simulink model "main"  (R2019a)
settings: Solver=ode45  StartTime=0.0  StopTime=simTime  FixedStep=Ts  RelTol=1e-3  EnableMultiTasking=on
values from neighbouring files (symbols this model uses):
  alfa1 = .2    (= 0.2)    [parameters.m]
  alfa2 = .2    (= 0.2)    [parameters.m]
  b1 = 0.1    [parameters.m]
  b2 = 0.1    [parameters.m]
  b3_nom = 0.1    [parameters.m]
  b4_nom = 0.1    [parameters.m]
  b5 = 0.1    [parameters.m]
  C = zeros(2,10); C(1,1) = 1; C(2,4) = 1    [parameters.m]
  C_D_Re_GNARC = C_C_Re    [init.m]
  D_D_Re_GNARC = D_C_Re    [init.m]
  DELTAS = cat(3,DELTAS,delta_c2d)    [dht.m]
  GAMMA = eye(10)    [parameters.m]
  initial_P = inmat.P_ss    [parameters.m]
  initial_probs = [1.0/N_hypos 1.0/N_hypos 1.0/N_hypos]    [dht.m]
  initial_state = [0,0,0,0,0,0,0,0,0,0]'    [parameters.m]
  k1 = 0.15    [parameters.m]
  k2 = (2.5-0.75)/2    (= 0.875)    [parameters.m]
  k3_nom = .1    (= 0.1)    [parameters.m]
  k4_nom = .1    (= 0.1)    [parameters.m]
  k5 = (2.5-0.9)/2    (= 0.8)    [parameters.m]
  Ks = cat(3,Ks,Li)    [dht.m]
  ks = [[2.0 2.0]; [1.0 1.75]; [2.0 1.25]]    [dht.m]
  m1 = 1    [parameters.m]
  m2 = 1    [parameters.m]
  m3 = 1    [parameters.m]
  m4 = 1    [parameters.m]
  PHIS = cat(3,PHIS,phi_c2d)    [dht.m]
  Qd = A_d*N(1:10, 11:20)    [parameters.m]
  Rd = R ./ Ts    [parameters.m]
  Sh_dets = cat(3,Sh_dets,det(Shtemp))    [dht.m]
  Sh_invs = cat(3,Sh_invs,inv(Shtemp))    [dht.m]
  simNo = 10    [parameters.m]    (also in qsimall.m = i)
  simTime = 300    [parameters.m]    (also in qsimall.m = 400)
  Ts = .001    (= 0.001)    [parameters.m]
undefined symbols (not defined in the file or in its folder): A_D_Re_GNARC, B_D_Re_GNARC, DELTA, PHI
libraries: simulink x4
settings Model: Creator=VAHiD  LastModifiedBy=revolt
settings DataIOCC: LimitDataPoints=on  SaveFormat=Array  SignalLoggingSaveFormat=ModelDataLogs  ReturnWorkspaceOutputs=off
settings OptimizationCC: ExpressionDepthLimit=2147483647  LifeSpan=inf
settings DebuggingCC: UnderspecifiedInitializationDetection=Classic  MergeDetectMultiDrivingBlocksExec=none  SolverPrmCheckMsg=warning  FcnCallInpInsideContextMsg=warning  StateNameClashWarn=warning  PregeneratedLibrarySubsystemCodeDiagnostic=none  SFUnexpectedBacktrackingDiag=warning  SFNoUnconditionalDefaultTransitionDiag=warning  SFExecutionAtInitializationDiag=none  ArithmeticOperatorsInVariantConditions=warning
settings HardwareCC: ProdBitPerPointer=32  ProdBitPerSizeT=32  ProdBitPerPtrDiffT=32  ProdLargestAtomicFloat=None  ProdIntDivRoundTo=Undefined  ProdEndianess=Unspecified  ProdWordSize=32  ProdHWDeviceType=32-bit Generic
settings ModelReferenceCC: PropagateSignalLabelsOutOfModel=off
settings SFSimCC: SimUseLocalCustomCode=off
settings RTWCC: RTWUseLocalCustomCode=off
settings CodeAppCC: StateflowObjectComments=on
settings GRTTargetCC: TargetLangStandard=C89/C90 (ANSI)  GeneratePreprocessorConditionals=Disable all  CombineOutputUpdateFcns=off  GRTInterface=on
settings ConfigComp: CovMetricSettings=dw  CovHtmlReporting=on  CovSaveCumulativeToWorkspaceVar=on  CovSaveSingleToWorkspaceVar=on  CovExternalEMLEnable=off

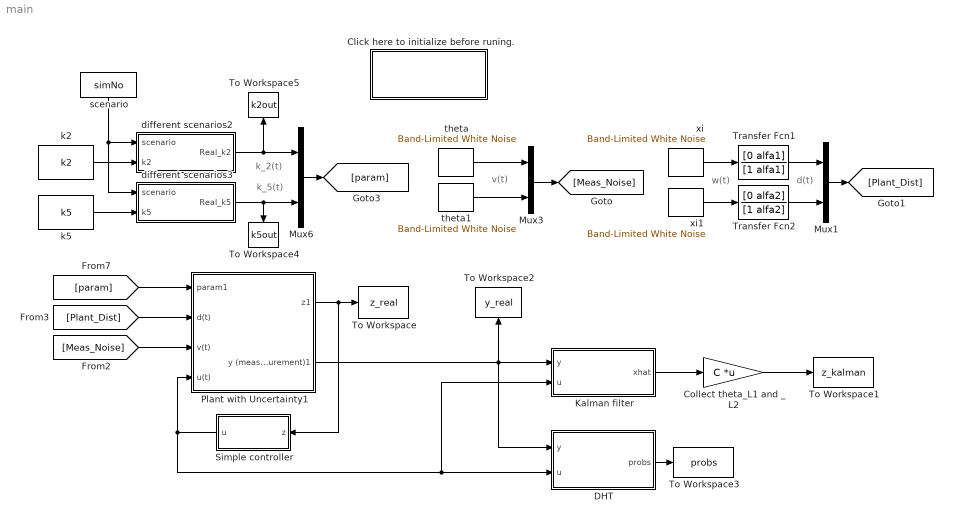
== system main ==
  note: w(t)
  note: v(t)
  note: d(t)
  note: k_2(t)
  note: k_5(t)
  Click here to initialize before runing. : Subsystem
      settings: OpenFcn=start_up
      mask Display: disp('Load\Parameters')
  Collect theta_L1 and _L2 : Gain  Gain=C  Multiplication=Matrix(K*u)
  DHT : Subsystem
  Kalman filter : Subsystem
  Mux1 : Mux  Inputs=2
  Mux3 : Mux  Inputs=2
  Mux6 : Mux  Inputs=2
  Plant with Uncertainty1 : Subsystem
  Simple controller : Subsystem
  To Workspace : ToWorkspace  VariableName=z_real  SaveFormat=Timeseries  SampleTime=-1
  To Workspace1 : ToWorkspace  VariableName=z_kalman  SaveFormat=Timeseries  SampleTime=-1
  To Workspace2 : ToWorkspace  VariableName=y_real  SaveFormat=Timeseries  SampleTime=-1
  To Workspace3 : ToWorkspace  VariableName=probs  SaveFormat=Timeseries  SampleTime=-1
  To Workspace4 : ToWorkspace  VariableName=k5out  SaveFormat=Timeseries  SampleTime=-1
  To Workspace5 : ToWorkspace  VariableName=k2out  SaveFormat=Timeseries  SampleTime=-1
  Transfer Fcn1 : TransferFcn  Numerator=[0 alfa1]  Denominator=[1 alfa1]
  Transfer Fcn2 : TransferFcn  Numerator=[0 alfa2]  Denominator=[1 alfa2]
  different scenarios2 : Subsystem
  different scenarios3 : Subsystem
  k2 : Constant  Value=k2
  k5 : Constant  Value=k5
  scenario : Constant  Value=simNo
  theta : simulink/Sources/Band-Limited White Noise  Cov=TH1  Ts=Ts  seed=1
  theta1 : simulink/Sources/Band-Limited White Noise  Cov=TH2  Ts=Ts  seed=2
  xi : simulink/Sources/Band-Limited White Noise  Cov=XI1  Ts=Ts  seed=3
  xi1 : simulink/Sources/Band-Limited White Noise  Cov=XI2  Ts=Ts  seed=4
  wires:
  Mux3/1 -> [Meas_Noise]
  theta/1 -> Mux3/1
  theta1/1 -> Mux3/2
  Mux1/1 -> [Plant_Dist]
  xi/1 -> Transfer Fcn1/1
  xi1/1 -> Transfer Fcn2/1
  Transfer Fcn1/1 -> Mux1/1
  Transfer Fcn2/1 -> Mux1/2
  scenario/1 -> different scenarios2/1(scenario), different scenarios3/1(scenario)
  k2/1 -> different scenarios2/2(k2)
  k5/1 -> different scenarios3/2(k5)
  different scenarios3/1(Real_k5) -> Mux6/2, To Workspace4/1
  different scenarios2/1(Real_k2) -> Mux6/1, To Workspace5/1
  Mux6/1 -> [param]
  [param] -> Plant with Uncertainty1/1(param1)
  [Plant_Dist] -> Plant with Uncertainty1/2(d(t))
  [Meas_Noise] -> Plant with Uncertainty1/3(v(t))
  Simple controller/1(u) -> Plant with Uncertainty1/4(u(t)), Kalman filter/2(u), DHT/2(u)
  Plant with Uncertainty1/2(y (measurement)1) -> DHT/1(y), Kalman filter/1(y), To Workspace2/1
  Kalman filter/1("xhat ") -> Collect theta_L1 and _L2/1
  Collect theta_L1 and _L2/1 -> To Workspace1/1
  Plant with Uncertainty1/1(z1) -> To Workspace/1, Simple controller/1(z)
  DHT/1(probs) -> To Workspace3/1

== system main/Click here to initialize before runing. ==

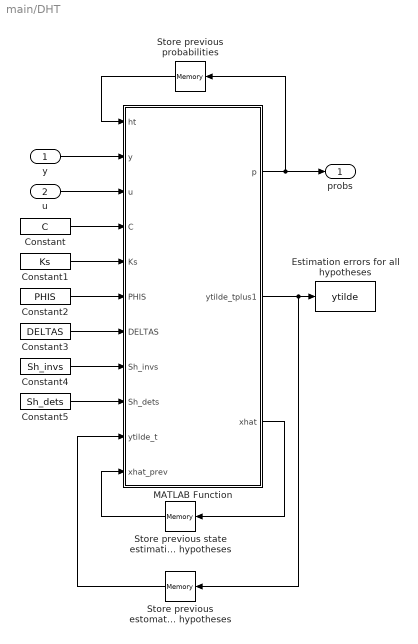
== system main/DHT ==
  y : Inport
  u : Inport  Port=2
  Constant : Constant  Value=C
  Constant1 : Constant  Value=Ks
  Constant2 : Constant  Value=PHIS
  Constant3 : Constant  Value=DELTAS
  Constant4 : Constant  Value=Sh_invs
  Constant5 : Constant  Value=Sh_dets
  Estimation errors for all hypotheses : ToWorkspace  VariableName=ytilde  SaveFormat=Timeseries  SampleTime=-1
  MATLAB Function : MATLAB Function  TreatAsAtomicUnit=on
  Store previous estomation errors for all hypotheses : Memory  InitialCondition=[zeros(2,1) zeros(2,1) zeros(2,1)]
  Store previous probabilities : Memory  InitialCondition=initial_probs
  Store previous state estimations for all hypotheses : Memory  InitialCondition=[initial_state initial_state initial_state]
  probs : Outport
  wires:
  MATLAB Function/1(p) -> probs/1, Store previous probabilities/1
  Store previous state estimations for all hypotheses/1 -> MATLAB Function/11(xhat_prev)
  Store previous probabilities/1 -> MATLAB Function/1(ht)
  y/1 -> MATLAB Function/2(y)
  u/1 -> MATLAB Function/3(u)
  Constant1/1 -> MATLAB Function/5(Ks)
  Constant2/1 -> MATLAB Function/6(PHIS)
  Constant3/1 -> MATLAB Function/7(DELTAS)
  Constant4/1 -> MATLAB Function/8(Sh_invs)
  Constant/1 -> MATLAB Function/4(C)
  Constant5/1 -> MATLAB Function/9(Sh_dets)
  MATLAB Function/3(xhat) -> Store previous state estimations for all hypotheses/1
  MATLAB Function/2(ytilde_tplus1) -> Store previous estomation errors for all hypotheses/1, Estimation errors for all hypotheses/1
  Store previous estomation errors for all hypotheses/1 -> MATLAB Function/10(ytilde_t)

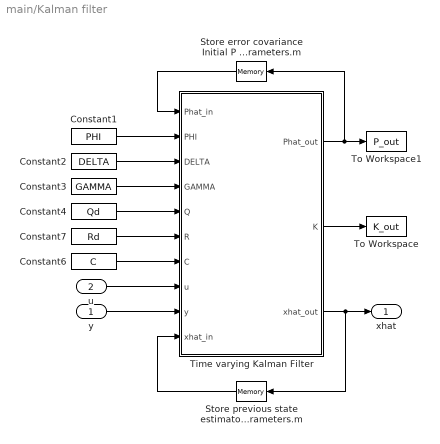
== system main/Kalman filter ==
  y : Inport
  u : Inport  Port=2
  Constant1 : Constant  Value=PHI
  Constant2 : Constant  Value=DELTA
  Constant3 : Constant  Value=GAMMA
  Constant4 : Constant  Value=Qd
  Constant6 : Constant  Value=C
  Constant7 : Constant  Value=Rd
  Store error covariance Initial P set in parameters.m : Memory  InitialCondition=initial_P
  Store previous state estimaton Initial state set in parameters.m : Memory  InitialCondition=initial_state
  Time varying Kalman Filter : MATLAB Function  TreatAsAtomicUnit=on
  To Workspace : ToWorkspace  VariableName=K_out  SaveFormat=Timeseries  SampleTime=-1
  To Workspace1 : ToWorkspace  VariableName=P_out  SaveFormat=Timeseries  SampleTime=-1
  "xhat " : Outport
  wires:
  u/1 -> Time varying Kalman Filter/8(u)
  Store previous state estimaton Initial state set in parameters.m/1 -> Time varying Kalman Filter/10(xhat_in)
  Time varying Kalman Filter/1(Phat_out) -> Store error covariance Initial P set in parameters.m/1, To Workspace1/1
  Store error covariance Initial P set in parameters.m/1 -> Time varying Kalman Filter/1(Phat_in)
  Constant3/1 -> Time varying Kalman Filter/4(GAMMA)
  Constant6/1 -> Time varying Kalman Filter/7(C)
  Constant7/1 -> Time varying Kalman Filter/6(R)
  y/1 -> Time varying Kalman Filter/9(y)
  Time varying Kalman Filter/3(xhat_out) -> "xhat "/1, Store previous state estimaton Initial state set in parameters.m/1
  Time varying Kalman Filter/2(K) -> To Workspace/1
  Constant2/1 -> Time varying Kalman Filter/3(DELTA)
  Constant1/1 -> Time varying Kalman Filter/2(PHI)
  Constant4/1 -> Time varying Kalman Filter/5(Q)

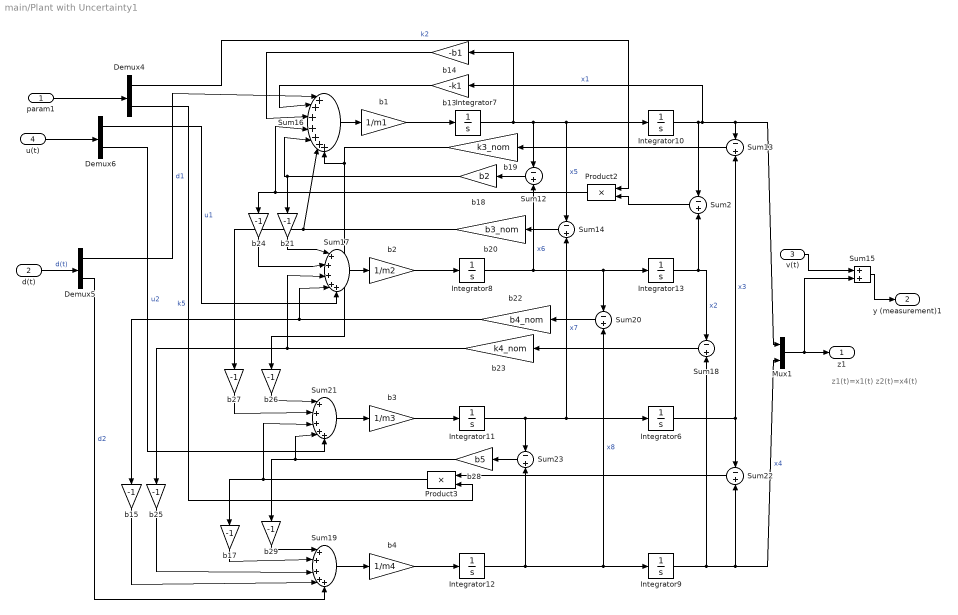
== system main/Plant with Uncertainty1 ==
  note: z1(t)=x1(t)
      | z2(t)=x4(t)
  param1 : Inport
  d(t) : Inport  Port=2
  v(t) : Inport  Port=3
  u(t) : Inport  Port=4
  Demux4 : Demux  Outputs=2
  Demux5 : Demux  Outputs=2
  Demux6 : Demux  Outputs=2
  Integrator{6..13} (8 alike) : Integrator
  Mux1 : Mux  Inputs=2
  Product2 : Product  SaturateOnIntegerOverflow=on  InputSameDT=on  OutDataTypeStr=Inherit: Same as first input
  Product3 : Product  SaturateOnIntegerOverflow=on  InputSameDT=on  OutDataTypeStr=Inherit: Same as first input
  Sum{2,12..14,18,20,22..23} (8 alike) : Sum  Inputs=-+  SaturateOnIntegerOverflow=on  InputSameDT=on  OutDataTypeStr=Inherit: Same as first input
  Sum15 : Sum  SaturateOnIntegerOverflow=on  InputSameDT=on  OutDataTypeStr=Inherit: Same as first input
  Sum16 : Sum  Inputs=|+++++++  SaturateOnIntegerOverflow=on  InputSameDT=on  OutDataTypeStr=Inherit: Same as first input
  Sum17 : Sum  Inputs=|+++++  SaturateOnIntegerOverflow=on  InputSameDT=on  OutDataTypeStr=Inherit: Same as first input
  Sum19 : Sum  Inputs=|+++++  SaturateOnIntegerOverflow=on  InputSameDT=on  OutDataTypeStr=Inherit: Same as first input
  Sum21 : Sum  Inputs=|+++++  SaturateOnIntegerOverflow=on  InputSameDT=on  OutDataTypeStr=Inherit: Same as first input
  b1 : Gain  Gain=1/m1  SaturateOnIntegerOverflow=on  OutDataTypeStr=Inherit: Same as input  ParamDataTypeStr=Inherit: Same as input
  b13 : Gain  Gain=-k1  SaturateOnIntegerOverflow=on  OutDataTypeStr=Inherit: Same as input  ParamDataTypeStr=Inherit: Same as input
  b14 : Gain  Gain=-b1  SaturateOnIntegerOverflow=on  OutDataTypeStr=Inherit: Same as input  ParamDataTypeStr=Inherit: Same as input
  b{15,17,21,24..27,29} (8 alike) : Gain  Gain=-1  SaturateOnIntegerOverflow=on  OutDataTypeStr=Inherit: Same as input  ParamDataTypeStr=Inherit: Same as input
  b18 : Gain  Gain=b2  SaturateOnIntegerOverflow=on  OutDataTypeStr=Inherit: Same as input  ParamDataTypeStr=Inherit: Same as input
  b19 : Gain  Gain=k3_nom  SaturateOnIntegerOverflow=on  OutDataTypeStr=Inherit: Same as input  ParamDataTypeStr=Inherit: Same as input
  b2 : Gain  Gain=1/m2  SaturateOnIntegerOverflow=on  OutDataTypeStr=Inherit: Same as input  ParamDataTypeStr=Inherit: Same as input
  b20 : Gain  Gain=b3_nom  SaturateOnIntegerOverflow=on  OutDataTypeStr=Inherit: Same as input  ParamDataTypeStr=Inherit: Same as input
  b22 : Gain  Gain=b4_nom  SaturateOnIntegerOverflow=on  OutDataTypeStr=Inherit: Same as input  ParamDataTypeStr=Inherit: Same as input
  b23 : Gain  Gain=k4_nom  SaturateOnIntegerOverflow=on  OutDataTypeStr=Inherit: Same as input  ParamDataTypeStr=Inherit: Same as input
  b28 : Gain  Gain=b5  SaturateOnIntegerOverflow=on  OutDataTypeStr=Inherit: Same as input  ParamDataTypeStr=Inherit: Same as input
  b3 : Gain  Gain=1/m3  SaturateOnIntegerOverflow=on  OutDataTypeStr=Inherit: Same as input  ParamDataTypeStr=Inherit: Same as input
  b4 : Gain  Gain=1/m4  SaturateOnIntegerOverflow=on  OutDataTypeStr=Inherit: Same as input  ParamDataTypeStr=Inherit: Same as input
  z1 : Outport
  y (measurement)1 : Outport  Port=2
  wires:
  Sum15/1 -> y (measurement)1/1
  v(t)/1 -> Sum15/1
  param1/1 -> Demux4/1
  Mux1/1 -> Sum15/2, z1/1
  d(t)/1 -> Demux5/1  "d(t)"
  u(t)/1 -> Demux6/1
  b25/1 -> Sum19/3
  b15/1 -> Sum19/4
  Demux5/2 -> Sum19/5  "d2"
  Integrator7/1 -> b14/1, Sum12/1, Integrator10/1, Sum14/1  "x5"
  Integrator10/1 -> b13/1, Sum13/1, Mux1/1, Sum2/1  "x1"
  Integrator8/1 -> Sum12/2, Integrator13/1, Sum20/1  "x6"
  Integrator11/1 -> Integrator6/1, Sum14/2, Sum23/1  "x7"
  Integrator12/1 -> Integrator9/1, Sum20/2, Sum23/2  "x8"
  Demux5/1 -> Sum16/1  "d1"
  b13/1 -> Sum16/2
  b14/1 -> Sum16/3
  Integrator13/1 -> Sum2/2, Sum18/1  "x2"
  Sum2/1 -> Product2/2
  Demux4/1 -> Product2/1  "k2"
  Sum12/1 -> b18/1
  b18/1 -> Sum16/5, b21/1
  Integrator6/1 -> Sum13/2, Sum22/1  "x3"
  Sum13/1 -> b19/1
  Sum14/1 -> b20/1
  b20/1 -> Sum16/6, b27/1
  Sum16/1 -> b1/1
  Product2/1 -> Sum16/4, b24/1
  Integrator9/1 -> Sum18/2, Sum22/2, Mux1/2  "x4"
  Sum18/1 -> b23/1
  b23/1 -> Sum17/3, b25/1
  Sum17/1 -> b2/1
  Sum20/1 -> b22/1
  b22/1 -> Sum17/4, b15/1
  b21/1 -> Sum17/1
  b24/1 -> Sum17/2
  Demux6/1 -> Sum17/5  "u1"
  Sum21/1 -> b3/1
  b19/1 -> Sum16/7, b26/1
  b26/1 -> Sum21/1
  b27/1 -> Sum21/2
  Sum22/1 -> Product3/1
  Product3/1 -> Sum21/3, b17/1
  Demux4/2 -> Product3/2  "k5"
  Sum23/1 -> b28/1
  b28/1 -> Sum21/4, b29/1
  Demux6/2 -> Sum21/5  "u2"
  Sum19/1 -> b4/1
  b17/1 -> Sum19/2
  b29/1 -> Sum19/1
  b1/1 -> Integrator7/1
  b2/1 -> Integrator8/1
  b3/1 -> Integrator11/1
  b4/1 -> Integrator12/1

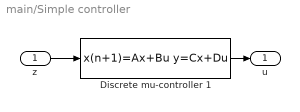
== system main/Simple controller ==
  z : Inport
  Discrete mu-controller 1 : DiscreteStateSpace  Description=disp('sss')  A=A_D_Re_GNARC  B=B_D_Re_GNARC  C=C_D_Re_GNARC  D=D_D_Re_GNARC  SampleTime=Ts
  u : Outport
  wires:
  z/1 -> Discrete mu-controller 1/1
  Discrete mu-controller 1/1 -> u/1

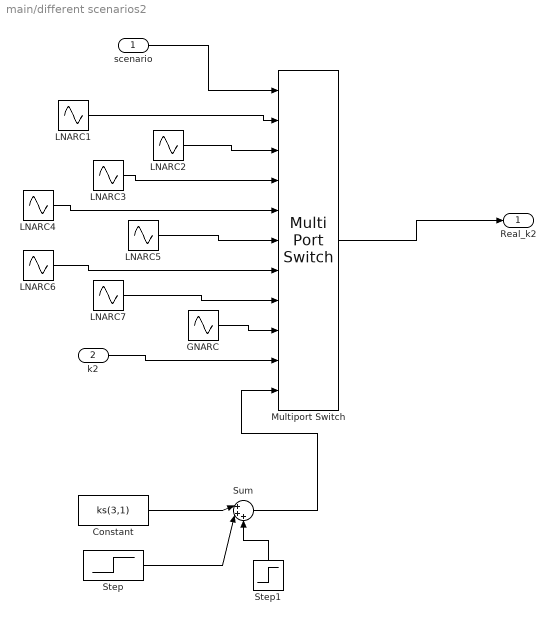
== system main/different scenarios2 ==
  scenario : Inport
  k2 : Inport  Port=2
  Constant : Constant  Value=ks(3,1)
  GNARC : Sin  Amplitude=.75  Bias=1  Frequency=2*pi/700  Phase=-pi/2  SampleTime=0
  LNARC1 : Sin  Amplitude=.875  Bias=1.625  Frequency=2*pi/700  Phase=-pi/2  SampleTime=0
  LNARC2 : Sin  Amplitude=.55/2  Bias=.775  Frequency=2*pi/700  Phase=-pi/2  SampleTime=0
  LNARC3 : Sin  Amplitude=.75/2  Bias=1.4250  Frequency=2*pi/700  Phase=-pi/2  SampleTime=0
  LNARC4 : Sin  Amplitude=.15/2  Bias=.325  Frequency=2*pi/100  Phase=-pi/2  SampleTime=0
  LNARC5 : Sin  Amplitude=.15  Bias=.55  Frequency=2*pi/100  Phase=-pi/2  SampleTime=0
  LNARC6 : Sin  Amplitude=.45/2  Bias=.925  Frequency=2*pi/700  Phase=-pi/2  SampleTime=0
  LNARC7 : Sin  Amplitude=.30  Bias=1.45  Frequency=2*pi/700  Phase=-pi/2  SampleTime=0
  Multiport Switch : MultiPortSwitch  Inputs=10
  Step : Step  Time=simTime / 3  After=ks(2,1) - ks(3,1)  SampleTime=0
  Step1 : Step  Time=simTime * 2/3  After=ks(1,1) - ks(2,1)  SampleTime=0
  Sum : Sum  Inputs=|+++
  Real_k2 : Outport
  wires:
  Multiport Switch/1 -> Real_k2/1
  scenario/1 -> Multiport Switch/1
  LNARC3/1 -> Multiport Switch/4
  LNARC6/1 -> Multiport Switch/7
  LNARC7/1 -> Multiport Switch/8
  LNARC5/1 -> Multiport Switch/6
  LNARC4/1 -> Multiport Switch/5
  LNARC1/1 -> Multiport Switch/2
  LNARC2/1 -> Multiport Switch/3
  k2/1 -> Multiport Switch/10
  GNARC/1 -> Multiport Switch/9
  Step/1 -> Sum/2
  Sum/1 -> Multiport Switch/11
  Constant/1 -> Sum/1
  Step1/1 -> Sum/3

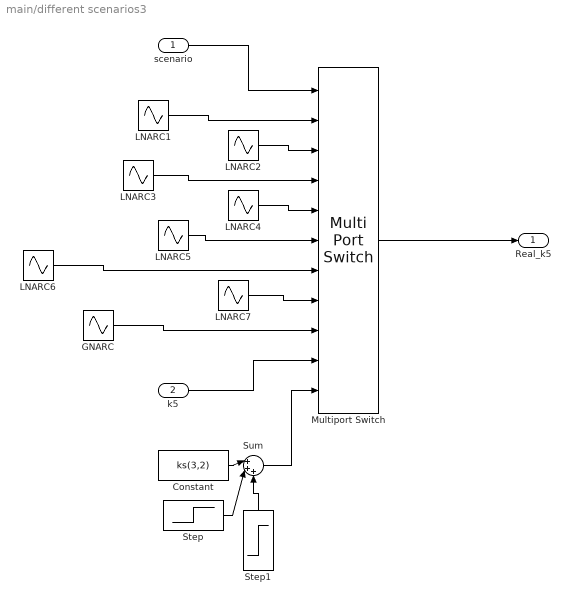
== system main/different scenarios3 ==
  scenario : Inport
  k5 : Inport  Port=2
  Constant : Constant  Value=ks(3,2)
  GNARC : Sin  Amplitude=1.6  Bias=1.8  Frequency=2*pi/700  Phase=-pi/2  SampleTime=0
  LNARC1 : Sin  Amplitude=.8  Bias=1.7  Frequency=2*pi/700  Phase=-3*pi/2  SampleTime=0
  LNARC2 : Sin  Amplitude=.8  Bias=2.6  Frequency=2*pi/700  Phase=-pi/2  SampleTime=0
  LNARC3 : Sin  Amplitude=.8  Bias=2.6  Frequency=2*pi/700  Phase=-pi/2  SampleTime=0
  LNARC{4..7} (4 alike) : Sin  Amplitude=.8  Bias=1  Frequency=2*pi/700  Phase=-pi/2  SampleTime=0
  Multiport Switch : MultiPortSwitch  Inputs=10
  Step : Step  Time=simTime/3  After=ks(2,2) - ks(3,2)  SampleTime=0
  Step1 : Step  Time=2*simTime /3  After=ks(1,2) - ks(2,2)  SampleTime=0
  Sum : Sum  Inputs=|+++
  Real_k5 : Outport
  wires:
  LNARC5/1 -> Multiport Switch/6
  LNARC7/1 -> Multiport Switch/8
  LNARC6/1 -> Multiport Switch/7
  LNARC3/1 -> Multiport Switch/4
  scenario/1 -> Multiport Switch/1
  k5/1 -> Multiport Switch/10
  GNARC/1 -> Multiport Switch/9
  LNARC1/1 -> Multiport Switch/2
  LNARC2/1 -> Multiport Switch/3
  LNARC4/1 -> Multiport Switch/5
  Multiport Switch/1 -> Real_k5/1
  Sum/1 -> Multiport Switch/11
  Step/1 -> Sum/2
  Constant/1 -> Sum/1
  Step1/1 -> Sum/3

== matlab function main/Kalman filter/Time varying Kalman Filter ==
  data: Phat_in input; PHI input; DELTA input; GAMMA input; Q input; R input; C input; u input; Phat_out output; K output; y input; xhat_out output; xhat_in input
function [Phat_out,K,xhat_out] = KF(Phat_in,PHI,DELTA,GAMMA,Q,R,C,u,    y,xhat_in)
% returns the predicted mean (=state) and covariance (-covariance of 
% predicted state estimate error) for a time step Ts, ref Fossen 2011 table 11.1

% PREDICTION
xbar = PHI * xhat_in + DELTA * u;
Pbar = PHI * Phat_in * PHI' + GAMMA * Q * GAMMA';

K = (Pbar * C') / (C * Pbar * C' + R);
xhat_out = xbar + K * (y - C * xbar);

I = eye(size(Pbar));
Phat_out = (I - K * C) * Pbar * (I - K * C)' + K * R * K';

end

== matlab function main/DHT/MATLAB Function ==
  data: ht input; y input; u input; C input; Ks input; PHIS input; DELTAS input; Sh_invs input; Sh_dets input; ytilde_t input; p output; ytilde_tplus1 output; xhat_prev input; xhat output
function [p,ytilde_tplus1,xhat] = DHT(ht,y,u,C,Ks,PHIS,DELTAS,Sh_invs,Sh_dets,ytilde_t,xhat_prev)
%
% ht        - the previous probabilities, h(t) = [h1(t) h2(t) h3(t)]
% y         - the measurement (2x1) at time t+1
% u         - the input value (2x1) at time t
% C,Ks,PHIS,DELTAS,Sh_invs,Sh_dets - loads of physical quantities
% ytilde_t  - the estimated error at time t, = [[error1], [error2], [error3]]
% xhat_prev - previous state estimates (10x3) at time t

N = length(ht);             % Number of hypotheses
ytilde_tplus1 = zeros(2,N); % 2 measurements
xhat = zeros(10,N);         % 10 states, 3 hypothesis
hs = zeros(N,1);            % Pre-allocate probability memory

% Obtain estimation predictions and probability "parts"
for i = 1:N    
    
    % Predict and correct state estimate for time t+1 wrt. quantities at time t
    xhat(:,i) = PHIS(:,:,i) * xhat_prev(:,i) + DELTAS(:,:,i) * u + Ks(:,:,i) * ytilde_t(:,i);
    
    % Update estimation error at time t+1 
    ytilde_tplus1(:,i) = y - C * xhat(:,i); % ytilde(t+1)
    
    % Calculate individual probabily elements (above the fraction) at time t+1
    hs(i) = exp(-0.5 * ytilde_tplus1(:,i)' * Sh_invs(:,:,i) * ytilde_tplus1(:,i) ) / sqrt( (2*pi)^2 * Sh_dets(i) );
end

% Calculate the sum of all the "probabilities"
htot = 0;
for i = 1:N
    htot = htot + hs(i)*ht(i);
end

% Calculate normalized probabilities
p = zeros(3,1);
for i = 1:N
    p(i) = (hs(i) * ht(i)) / htot;
end

% Avoid numerical rounding errors if one probability gets too large / the others
% gets too small. Without this control, the DHT caused the hypothesis 
% that was allowed to be most likely for a long period of time to be the only
% one that were set to true for the rest of the simulation. Since MATLAB
% operates with a certain precision, the other hypotheses' probabilities were
% set to zero, causing them to never become true.
boundary = 0.999999;
for i = 1:N
    if p(i) > boundary
        p(i) = boundary;
        p(p<boundary) = (1 - boundary)/2; % They are so small that they can just be set to be equal
        break
    end
end
